simulink library "upfir"  (R2022b)
settings: Solver=VariableStepAuto  StartTime=0.0  StopTime=10.0  RelTol=1e-3
undefined symbols (not defined in the file or in its folder): numChannels, polyLen
libraries: FeaturePath x1
settings Model: Creator=jb10849  LastModifiedBy=kl13806
settings SolverCC: AlgebraicLoopSolver=TrustRegion
settings DebuggingCC: UnconnectedInputMsg=warning  UnconnectedOutputMsg=warning  UnconnectedLineMsg=warning  SFMachineParentedDataDiag=warning  ArithmeticOperatorsInVariantConditions=warning
settings ModelReferenceCC: EnableRefExpFcnMdlSchedulingChecks=on
settings SFSimCC: SimUseLocalCustomCode=off  CustomCodeUndefinedFunction=UseInterfaceOnly
settings RTWCC: RTWUseLocalCustomCode=off  DLArmComputeVersion=19.05
settings CodeAppCC: StateflowObjectComments=on

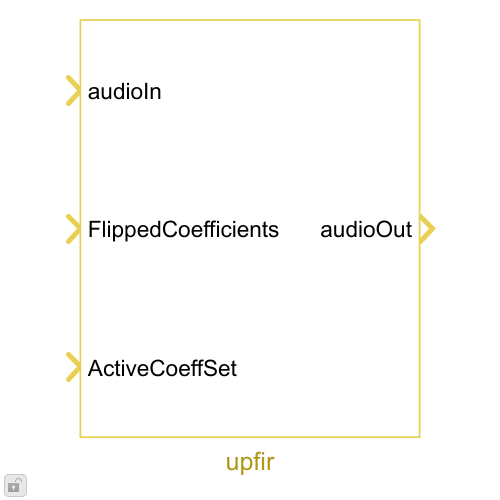
[thumbnail: Simulink's stored preview of the top-level diagram]
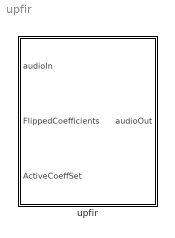
== system upfir ==
  upfir : Subsystem  mask{interp_factor=4}
      mask prompts: interp_factor "Interpolation Factor"
      mask help: Enter an even interpolation factor

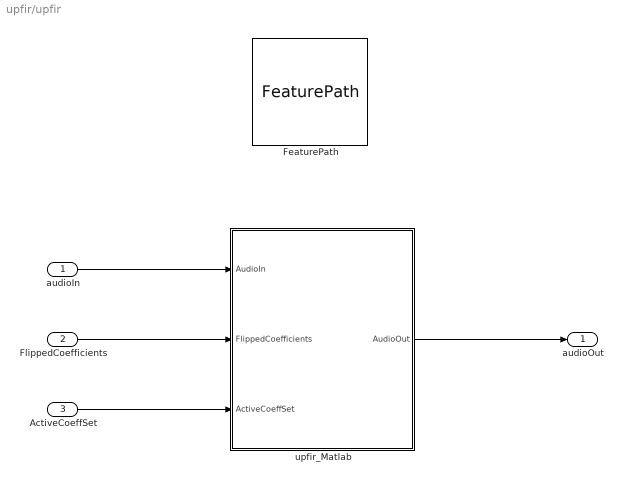
== system upfir/upfir ==
  audioIn : Inport
  FlippedCoefficients : Inport  Port=2
  ActiveCoeffSet : Inport  Port=3
  FeaturePath : FeaturePath/FeaturePath  FeatureName=upfir  IsGroup=on  GroupNumber=-1  IsModule=off  TriggerInit=[465 -26 580 81]
  upfir_Matlab : Subsystem
  audioOut : Outport  VectorParamsAs1DForOutWhenUnconnected=off
  wires:
  FlippedCoefficients/1 -> upfir_Matlab/2(FlippedCoefficients)
  ActiveCoeffSet/1 -> upfir_Matlab/3(ActiveCoeffSet)
  audioIn/1 -> upfir_Matlab/1(AudioIn)
  upfir_Matlab/1(AudioOut) -> audioOut/1

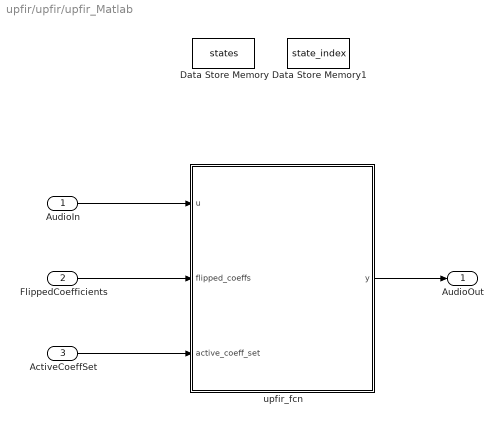
== system upfir/upfir/upfir_Matlab ==
  AudioIn : Inport
  FlippedCoefficients : Inport  Port=2
  ActiveCoeffSet : Inport  Port=3
  Data Store Memory : DataStoreMemory  DataStoreName=states  InitialValue=single(zeros(polyLen + 2, numChannels))  ShowAdditionalParam=off  OutDataTypeStr=single
  Data Store Memory1 : DataStoreMemory  DataStoreName=state_index  ShowAdditionalParam=off  OutDataTypeStr=int32
  upfir_fcn : MATLAB Function  TreatAsAtomicUnit=on
  AudioOut : Outport  VectorParamsAs1DForOutWhenUnconnected=off
  wires:
  FlippedCoefficients/1 -> upfir_fcn/2(flipped_coeffs)
  ActiveCoeffSet/1 -> upfir_fcn/3(active_coeff_set)
  AudioIn/1 -> upfir_fcn/1(u)
  upfir_fcn/1(y) -> AudioOut/1

== matlab function upfir/upfir_Matlab/upfir_fcn ==
  data: u input; y output; flipped_coeffs input; active_coeff_set input; interp_factor parameter; states data_store_memory; state_index data_store_memory
function y = UpFIR(u, flipped_coeffs, active_coeff_set, interp_factor)
% UP-FIR implements up-sampling by an integer factor followed by a FIR 
% filter. The back-to-back processing is accomplished using an efficient 
% polyphase implementation. Let ‘I’ represent the up-sampling factor.  
% Only the first BlockSize/I input samples are used and all BlockSize 
% output samples are generated.  The block supports multiple channels, 
% with each channel sharing the same set of filter coefficients.

% Extract configuration information from inputs
[taps, ~] = size(flipped_coeffs);
[framesize_dec, num_channels] = size(u);
frame_size = framesize_dec*interp_factor;
polyLen = taps/interp_factor;

% Initialize variables
global  states;
global state_index;

% Set correct data types
filter_length = int32(taps);
frame_size = uint32(frame_size);
num_channels = uint32(num_channels);
active_coeff_set = uint32(active_coeff_set);
interpolation_factor = int32(interp_factor);
polyLen = int32(polyLen);
% Call upfir function
y = upfir(u, frame_size, num_channels, states, filter_length, state_index, flipped_coeffs, active_coeff_set, interpolation_factor, polyLen);

end

function y = upfir(u, framesize, numChannels, states2, filterLength, stateIndex2, coeffs, activeCoeffSet, interp_factor, polylen)
% If target == codegen, generate warning if no CRL found
coder.replace('-warnifnoreplacement');
% States
global state_index;
global  states;

%Initialize variables
y = single(zeros(framesize,numChannels));
interp_factor = uint32(interp_factor);
% Process all channel inputs
for channel=1:numChannels
    %Initialize variables
    stateIndex = state_index;
    state= states(:,channel);
    coeff=coeffs(:,activeCoeffSet(channel)+1);
    coeffIndex=0;
    inSample=0;
    % Process each sample
    for sample=1:framesize
        phase=rem(sample-1, interp_factor);
        if (phase == 0)
            state(stateIndex+1)=u(inSample+1,channel);
            inSample=inSample+1;
            stateIndex=stateIndex+1;
            if (stateIndex == polylen)
                stateIndex=int32(0);
            end
        end
        % Polyphase implementation
        accum=single(0);
        for i=1:polylen
            accum=accum+state(stateIndex + 1) * coeff(coeffIndex+1);
            coeffIndex=coeffIndex+1;
            if (coeffIndex == filterLength)
                coeffIndex=0;
            end

            stateIndex=stateIndex+1;
            if (stateIndex == polylen)
                stateIndex=int32(0);
            end
        end
        y(sample, channel)=accum;
    end % sample loop
    states(:,channel) = state;
end
% update the state_index
state_index=stateIndex;
end
